simulink model "Model"  (R2018a)
settings: Solver=VariableStepAuto  StartTime=0.0  StopTime=1  RelTol=1e-3
values from neighbouring files (symbols this model uses):
  Gc = [1000 1000 1000 1000 400]    [BypassDiode.m]    (also in PVcell.m = 400; UIModulaG.m = i*200; UIModulaT.m = 1000; Untitled6.m = [Gc1 Gc1 Gc2 Gc2])
  Tc = [30 30 30 30 30]    [BypassDiode.m]    (also in UIModulaG.m = 25; UIModulaT.m = -50+i*25; Untitled6.m = [Tc1 Tc1 Tc2 Tc2]; kolf.m = [Tc2 Tc2 Tc2 Tc2])
libraries: simulink x2
settings Model: Creator=User  LastModifiedBy=User

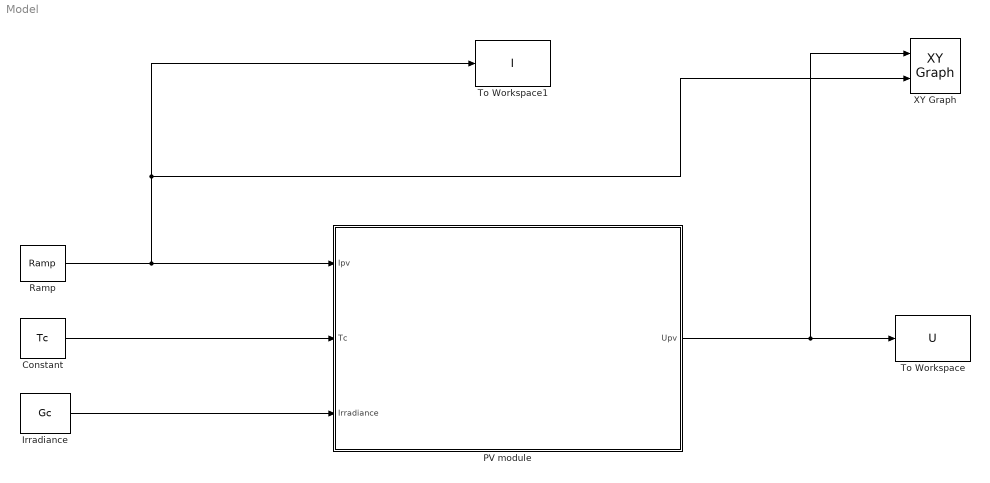
== system Model ==
  Constant : Constant  Value=Tc
  "Irradiance " : Constant  Value=Gc
  PV module : Subsystem  mask{Isc_ref=3.11, Uoc_ref=21.8, Imp=2.88, Ump=17, Rs=0.45, Rp=310, Ns=36, PV_mat=Si, PV_teh=Si-poly, Diode=on}
      mask prompts: Isc_ref "Short-circuit current [A]"; Uoc_ref "Open-circuit voltage [V]"; Imp "Current at Pmax [A]"; Ump "Voltage at Pmax [V]"; Rs "Series resistance of the PV module [Ohms]"; Rp "Shunt resistance of the PV module [Ohms]"; Ns "Number of cells connected in series"; PV_mat "Material"; PV_teh "PV cell technology"; Diode "Bypass diode?"
      mask init:
      | %============================================================
      | % Originator:
      | %   University of Banja Luka
      | %   Faculty of Electrical Engineering 
      | %   Department of Electrical Power Engineering
      | %   
      | % History:
      | %   16.1.2016. Version 1 
      | %============================================================
      | % Calculation of PV module parameters
      | %------------------------------------------------------------
      | k       = 1.381e-23; % [J/K] Boltzmann constant
      | q       = 1.602e-19; % [C] Charge of an electron
      | Tc_ref  = 25;        % [C] PV cell temperature at STC
      | G_ref   = 1000;      % [W/m2] Irradiance at STC
      | mi_sc   = 0.0013;    % [A/C] Temperature coefficient of the 
      |                      %       short circuit current     
      | 
      | % eps_g - [eV] Band gap of the material
      | switch PV_mat
      |     case 1
      |         eps_g = 1.12;
      |     case 2
      |         eps_g = 1.42;
      |     case 3
      |         eps_g = 1.50;
      |     case 4
      |         eps_g = 1.35;
      | end
      | 
      | % A - Ideality factor
      | switch PV_teh
      |     case 1
      |         A = 1.2;
      |     case 2
      |         A = 1.3;
      |     case 3
      |         A = 1.8;
      |     case 4
      |         A = 3.3;
      |     case 5
      |         A = 5;
      |     case 6
      |         A = 1.5;
      |     case 7
      |         A = 1.5;
      |     case 8
      |         A = 1.3;
      | end
      | %===========================================================
      mask TypeOptions PV_mat: Si | GaAs | CdTe | InP
      mask TypeOptions PV_teh: Si-mono | Si-poly | a-Si-H | a-Si-H tandem | a-Si-H triple | CdTe | CTs | AsGa
      mask Display:
      | plot([0.35 0.45],[0.3 0.7]);
      | plot([0.45 0.55],[0.3 0.7]);
      | plot([0.55 0.65],[0.3 0.7]);
      | plot([0.65 0.75],[0.3 0.7]);
      | plot([0.35 0.65],[0.3 0.3]);
      | plot([0.375 0.675],[0.4 0.4]);
      | plot([0.4 0.7],[0.5 0.5]);
      | plot([0.425 0.725],[0.6 0.6]);
      | plot([0.45 0.75],[0.7 0.7]);
      | text(0.5,0.9,'PV module','horizontalAlignment', 'center');
      | text(0.85,0.1,'ETF BL','horizontalAlignment', 'center');
  Ramp : simulink/Sources/Ramp  slope=1  start=0  InitialOutput=0
  To Workspace : ToWorkspace  VariableName=U  SampleTime=-1
  To Workspace1 : ToWorkspace  VariableName=I  SampleTime=-1
  XY Graph : simulink/Sinks/XY Graph  xmin=0  xmax=22  ymin=0  ymax=3.2  st=-1
  wires:
  Ramp/1 -> XY Graph/2, To Workspace1/1, PV module/1(Ipv)
  Constant/1 -> PV module/2(Tc)
  "Irradiance "/1 -> PV module/3(Irradiance)
  PV module/1(Upv) -> XY Graph/1, To Workspace/1

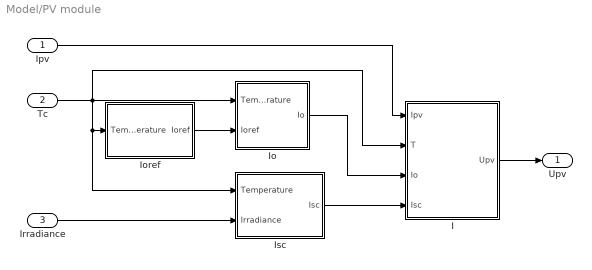
== system Model/PV module ==
  Ipv : Inport
  Tc : Inport  Port=2
  Irradiance : Inport  Port=3
  I : Subsystem
  Io : Subsystem
  Ioref : Subsystem
  Isc : Subsystem
  Upv : Outport
  wires:
  I/1(Upv) -> Upv/1
  Ipv/1 -> I/1(Ipv)
  Irradiance/1 -> Isc/2(Irradiance)
  Tc/1 -> I/2(T), Isc/1(Temperature), Ioref/1(Temperature), Io/1(Temperature)
  Io/1(Io) -> I/3(Io)
  Isc/1(Isc) -> I/4(Isc)
  Ioref/1(Ioref) -> Io/2(Ioref)

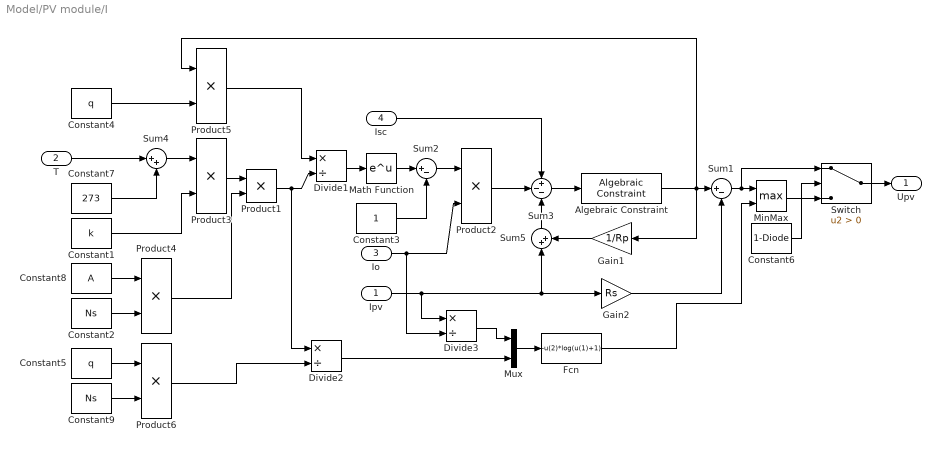
== system Model/PV module/I ==
  Ipv : Inport
  T : Inport  Port=2
  Io : Inport  Port=3
  Isc : Inport  Port=4
  Algebraic Constraint : AlgebraicConstraint
  Constant1 : Constant  Value=k
  Constant2 : Constant  Value=Ns
  Constant3 : Constant
  Constant4 : Constant  Value=q
  Constant5 : Constant  Value=q
  Constant6 : Constant  Value=1-Diode
  Constant7 : Constant  Value=273
  Constant8 : Constant  Value=A
  Constant9 : Constant  Value=Ns
  Divide1 : Product  Inputs=*/
  Divide2 : Product  Inputs=*/
  Divide3 : Product  Inputs=*/
  Fcn : Fcn  Expr=-u(2)*log(u(1)+1)
  Gain1 : Gain  Gain=1/Rp
  Gain2 : Gain  Gain=Rs
  Math Function : Math  SaturateOnIntegerOverflow=on
  MinMax : MinMax  Function=max  Inputs=2
  Mux : Mux  Inputs=2
  Product{1..6} (6 alike) : Product  RndMeth=Zero
  Sum1 : Sum  Inputs=|+-
  Sum2 : Sum  Inputs=|+-
  Sum3 : Sum  Inputs=+--
  Sum4 : Sum  Inputs=|++
  Sum5 : Sum  Inputs=|++
  Switch : Switch  Criteria=u2 > Threshold
  Upv : Outport
  wires:
  Product6/1 -> Divide2/2
  Constant9/1 -> Product6/2
  Constant5/1 -> Product6/1
  Constant6/1 -> Switch/2
  MinMax/1 -> Switch/3
  Switch/1 -> Upv/1
  Fcn/1 -> MinMax/2
  Sum1/1 -> Switch/1, MinMax/1
  Divide2/1 -> Mux/2
  Divide3/1 -> Mux/1
  Mux/1 -> Fcn/1
  Gain2/1 -> Sum1/2
  Gain1/1 -> Sum5/2
  Sum5/1 -> Sum3/3
  Ipv/1 -> Gain2/1, Sum5/1, Divide3/1
  Algebraic Constraint/1 -> Sum1/1, Product5/1, Gain1/1
  Sum3/1 -> Algebraic Constraint/1
  Isc/1 -> Sum3/1
  Product2/1 -> Sum3/2
  Io/1 -> Divide3/2, Product2/2
  Sum2/1 -> Product2/1
  Constant3/1 -> Sum2/2
  Math Function/1 -> Sum2/1
  Divide1/1 -> Math Function/1
  Product5/1 -> Divide1/1
  Constant4/1 -> Product5/2
  Product1/1 -> Divide2/1, Divide1/2
  Product4/1 -> Product1/2
  Constant2/1 -> Product4/2
  Constant8/1 -> Product4/1
  Product3/1 -> Product1/1
  Constant1/1 -> Product3/2
  Sum4/1 -> Product3/1
  Constant7/1 -> Sum4/2
  T/1 -> Sum4/1

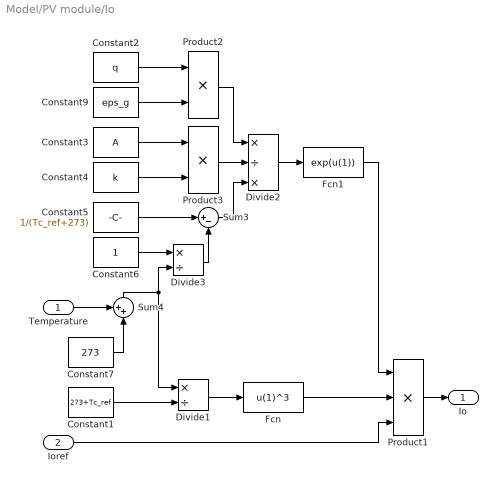
== system Model/PV module/Io ==
  Temperature : Inport
  Ioref : Inport  Port=2
  Constant1 : Constant  Value=273+Tc_ref
  Constant2 : Constant  Value=q
  Constant3 : Constant  Value=A
  Constant4 : Constant  Value=k
  Constant5 : Constant  Value=1/(Tc_ref+273)
  Constant6 : Constant
  Constant7 : Constant  Value=273
  Constant9 : Constant  Value=eps_g
  Divide1 : Product  Inputs=*/
  Divide2 : Product  Inputs=*/*
  Divide3 : Product  Inputs=*/
  Fcn : Fcn  Expr=u(1)^3
  Fcn1 : Fcn  Expr=exp(u(1))
  Product1 : Product  Inputs=3  RndMeth=Zero
  Product2 : Product  RndMeth=Zero
  Product3 : Product  RndMeth=Zero
  Sum3 : Sum  Inputs=|+-
  Sum4 : Sum  Inputs=++|
  Io : Outport
  wires:
  Constant1/1 -> Divide1/2
  Sum4/1 -> Divide1/1, Divide3/2
  Product1/1 -> Io/1
  Ioref/1 -> Product1/3
  Fcn/1 -> Product1/2
  Fcn1/1 -> Product1/1
  Divide2/1 -> Fcn1/1
  Sum3/1 -> Divide2/3
  Divide3/1 -> Sum3/2
  Divide1/1 -> Fcn/1
  Constant6/1 -> Divide3/1
  Temperature/1 -> Sum4/1
  Constant7/1 -> Sum4/2
  Constant5/1 -> Sum3/1
  Product3/1 -> Divide2/2
  Product2/1 -> Divide2/1
  Constant4/1 -> Product3/2
  Constant3/1 -> Product3/1
  Constant9/1 -> Product2/2
  Constant2/1 -> Product2/1

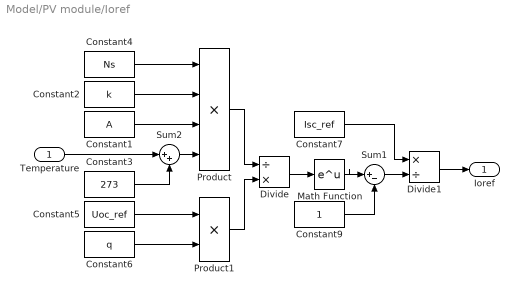
== system Model/PV module/Ioref ==
  Temperature : Inport
  Constant1 : Constant  Value=A
  Constant2 : Constant  Value=k
  Constant3 : Constant  Value=273
  Constant4 : Constant  Value=Ns
  Constant5 : Constant  Value=Uoc_ref
  Constant6 : Constant  Value=q
  Constant7 : Constant  Value=Isc_ref
  Constant9 : Constant
  Divide : Product  Inputs=/*
  Divide1 : Product  Inputs=*/
  Math Function : Math  SaturateOnIntegerOverflow=on
  Product : Product  Inputs=4  RndMeth=Zero
  Product1 : Product  RndMeth=Zero
  Sum1 : Sum  Inputs=|+-
  Sum2 : Sum  Inputs=|++
  Ioref : Outport
  wires:
  Constant2/1 -> Product/2
  Divide1/1 -> Ioref/1
  Constant7/1 -> Divide1/1
  Sum1/1 -> Divide1/2
  Constant9/1 -> Sum1/2
  Math Function/1 -> Sum1/1
  Divide/1 -> Math Function/1
  Constant6/1 -> Product1/2
  Constant5/1 -> Product1/1
  Product1/1 -> Divide/2
  Product/1 -> Divide/1
  Constant4/1 -> Product/1
  Constant1/1 -> Product/3
  Sum2/1 -> Product/4
  Constant3/1 -> Sum2/2
  Temperature/1 -> Sum2/1

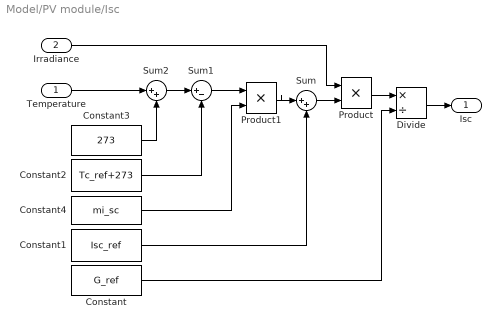
== system Model/PV module/Isc ==
  Temperature : Inport
  Irradiance : Inport  Port=2
  Constant : Constant  Value=G_ref
  Constant1 : Constant  Value=Isc_ref
  Constant2 : Constant  Value=Tc_ref+273
  Constant3 : Constant  Value=273
  Constant4 : Constant  Value=mi_sc
  Divide : Product  Inputs=*/
  Product : Product  RndMeth=Zero
  Product1 : Product  RndMeth=Zero
  Sum : Sum  Inputs=|++
  Sum1 : Sum  Inputs=|+-
  Sum2 : Sum  Inputs=|++
  Isc : Outport
  wires:
  Constant4/1 -> Product1/2
  Sum1/1 -> Product1/1
  Temperature/1 -> Sum2/1
  Divide/1 -> Isc/1
  Irradiance/1 -> Product/1
  Constant3/1 -> Sum2/2
  Constant2/1 -> Sum1/2
  Sum2/1 -> Sum1/1
  Product1/1 -> Sum/1
  Constant1/1 -> Sum/2
  Sum/1 -> Product/2
  Constant/1 -> Divide/2
  Product/1 -> Divide/1
